simulink model "SarImageFormation"  (Simulink 8.3)
settings: Solver=FixedStepDiscrete  StartTime=0.0  StopTime=0  RelTol=1e-3
model workspace: external: MAT-File SarImageWorkspace.mat (data not in the file)
values from neighbouring files (symbols this model uses):
  m = uicontextmenu('Parent',fig)    [HelperCreateParamTuningUI.m]    (also in HelperMeasureGroupDelay.m = length(p))
  mc = getappdata(uihandle,'midicontrol')    [HelperCreateParamTuningUI.m]
undefined symbols (not defined in the file or in its folder): dkx, fastTimeFilter, ic, jet, k, ku0, kxMin, kxs, magnitude, n, Newton, nInterpSidelobes, nx, Raphson, sRaw, uc, Xc
libraries: dspxfrm3 x4, dspsnks4 x2, dspmathops x2, dspSarDemoLib x2, dspsigops x1, dspmtrx3 x1, dspmisc x1, simulink x1
CloseFcn:
  | if exist('idxout','var') clear idxout; end
  | if exist('sarImage','var') clear sarImage; end
  | sarHandles=findobj('type','figure');
  | for idxh=1:length(sarHandles)
  |     if ~isempty(sarHandles(idxh)) && strcmp(get(sarHandles(idxh), 'UserData'),'SarDemoPlot')
  |        close(sarHandles(idxh));
  |     end
  | end
  | clear sarHandles;
  | clear idxh;
settings Model: FPTRunName=Active  Creator=The MathWorks Inc.  ExtModeAutoUpdateStatusClock=off
settings DataIOCC: SaveOutput=off  SaveTime=off
settings OptimizationCC: InlineParams=on  ExpressionDepthLimit=2147483647  InitFltsAndDblsToZero=on  OptimizeModelRefInitCode=on  LifeSpan=1
settings DebuggingCC: MultiTaskDSMMsg=warning  MultiTaskCondExecSysMsg=none  ParameterPrecisionLossMsg=none  FcnCallInpInsideContextMsg=UseLocalSettings  StrictBusMsg=None
settings HardwareCC: TargetHWDeviceType=32-bit Generic
settings SFSimCC: SimParseCustomCode=off
settings RTWCC: SystemTargetFile=ert.tlc  TemplateMakefile=ert_default_tmf  Description=Real-Time Workshop Embedded Coder (no auto configuration)  ProcessScript=ert_make_rtw_hook  IncludeERTFirstTime=on
settings CodeAppCC: IgnoreCustomStorageClasses=off  CustomSymbolStrType=$N$R$M  InternalIdentifier=Classic
settings ERTTargetCC: TargetFcnLib=ansi_tfl_tmw.mat  MultiwordLength=2048  GenerateSampleERTMain=on  MatFileLogging=on  ERTCustomFileTemplate=example_file_process.tlc  ConvertIfToSwitch=off  SuppressUnreachableDefaultCases=off

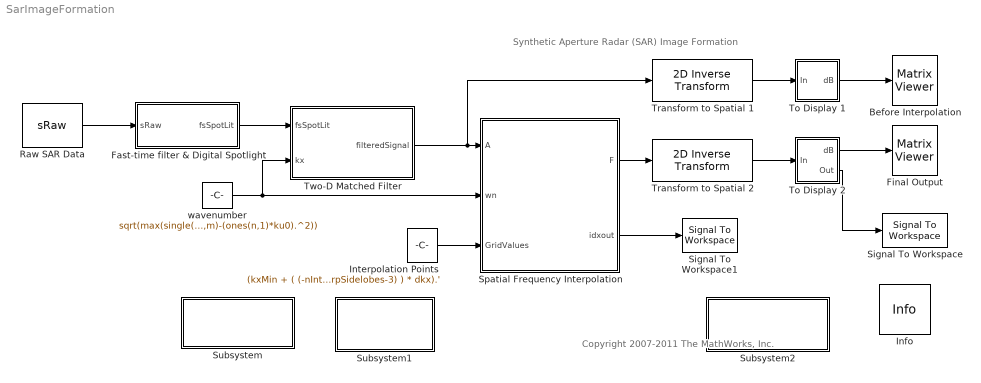
== system SarImageFormation ==
  note: Copyright 2007-2011 The MathWorks, Inc.
  note: Synthetic Aperture Radar (SAR) Image Formation
  Before Interpolation : dspsnks4/Matrix Viewer  ImageParams=off  CMapStr=jet(256)  AxisColorbar=on  AxisParams=off  AxisOrigin=Upper left corner  XLabel=Cross-range  YLabel=Range  ZLabel=Magnitude (dB)  FigPos=[5 300 500 420]  AxisZoom=off
      settings: YMin=0  YMax=60
  Fast-time filter & Digital Spotlight : Subsystem
  Final Output : dspsnks4/Matrix Viewer  ImageParams=off  CMapStr=jet(256)  AxisColorbar=on  AxisParams=off  AxisOrigin=Upper left corner  XLabel=Cross-range  YLabel=Range  ZLabel=Magnitude (dB)  FigPos=[510 300 500 420]  AxisZoom=off
      settings: YMin=0  YMax=60
  Info : dspmisc/Info  SystemSampleTime=-1
  Interpolation Points : Constant  Value=(kxMin + ( (-nInterpSidelobes-2):(nx-nInterpSidelobes-3) ) * dkx).'  VectorParams1D=off  SampleTime=Inf
  Raw SAR Data : Constant  Value=sRaw  VectorParams1D=off  SampleTime=1
  Signal To Workspace : SignalToWorkspace  VariableName=sarImage
      settings: CopyFcn=dspblkcopystw(gcbh);  Save2DSignal=3-D array (concatenate along third dimension)
  Signal To Workspace1 : SignalToWorkspace  VariableName=idxout
      settings: CopyFcn=dspblkcopystw(gcbh);  Save2DSignal=3-D array (concatenate along third dimension)
  Spatial Frequency Interpolation : MATLAB Function  TreatAsAtomicUnit=on
  Subsystem : Subsystem
      settings: OpenFcn=|
      | imagesc(20*log10(fftshift(abs(dspmodelvar(bdroot,'sRaw')))));
      | colorbar;
      | ylabel('Samples');xlabel('Pulses'); title('Spotlight SAR Returns')
      | set(gcf,'UserData','SarDemoPlot');
      mask Display: disp('Display raw\nSAR data (sRaw)')
  Subsystem1 : Subsystem
      settings: OpenFcn=|
      | imagesc(20*log10(abs(dspmodelvar(bdroot,'finalImage').')),[0 60]);
      | colorbar;
      | title('Truth image from MATLAB');
      | set(gcf,'UserData','SarDemoPlot');
      mask Display: disp('Display Truth\nSAR image')
  Subsystem2 : Subsystem
      settings: OpenFcn=|
      | if (exist('idxout','var')),                                        contourf(idxout,50);                                       cb=colorbar;                                                   xlabel('Cross-range');                                     ylabel('Range in source image');                     title('Interpolation Pattern');                            ylabel(cb,'Range in destination image');          clear('cb');
      |      set(gcf,'UserData','SarDemoPlot');            else                                                                     uiwait(errordlg('Data not found in workspace - run demo model.','DSP System Toolbox Demo Error','modal'));    end
      mask Display: disp('Display Interpolation\nPattern (idxout)')
  To Display 1 : Subsystem
  To Display 2 : Subsystem
  Transform to Spatial 1 : dspSarDemoLib/2D Inverse Transform
  Transform to Spatial 2 : dspSarDemoLib/2D Inverse Transform
  Two-D Matched Filter : Subsystem
  wavenumber : Constant  Value=sqrt(max(single(0), 4*(k.').^2*ones(1,m)-(ones(n,1)*ku0).^2))  VectorParams1D=off  SampleTime=Inf
  wires:
  Raw SAR Data/1 -> Fast-time filter & Digital Spotlight/1(sRaw)
  wavenumber/1 -> Spatial Frequency Interpolation/2(wn), Two-D Matched Filter/2(kx)
  To Display 2/1(dB) -> Final Output/1
  Interpolation Points/1 -> Spatial Frequency Interpolation/3(GridValues)
  Fast-time filter & Digital Spotlight/1(fsSpotLit) -> Two-D Matched Filter/1(fsSpotLit)
  Spatial Frequency Interpolation/1(F) -> Transform to Spatial 2/1
  Spatial Frequency Interpolation/2(idxout) -> Signal To Workspace1/1
  Transform to Spatial 2/1 -> To Display 2/1(" In")
  To Display 2/2(Out) -> Signal To Workspace/1
  Two-D Matched Filter/1(filteredSignal) -> Spatial Frequency Interpolation/1(A), Transform to Spatial 1/1
  Transform to Spatial 1/1 -> To Display 1/1(In)
  To Display 1/1(dB) -> Before Interpolation/1

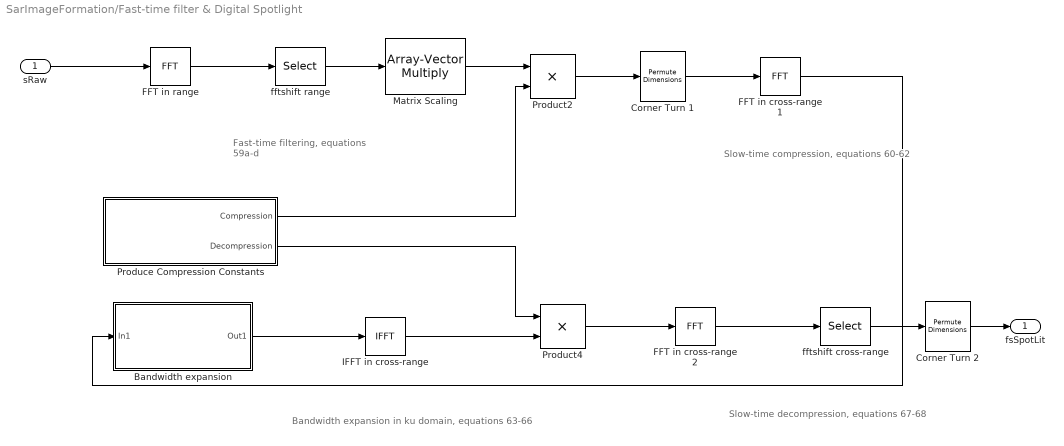
== system SarImageFormation/Fast-time filter & Digital Spotlight ==
  note: Fast-time filtering,
      | equations 59a-d
  note: Slow-time compression, equations 60-62
  note: Bandwidth expansion in ku domain, equations 63-66
  note: Slow-time decompression, equations 67-68
  sRaw : Inport
  Bandwidth expansion : Subsystem
  Corner Turn 1 : PermuteDimensions
  Corner Turn 2 : PermuteDimensions
  FFT in cross-range 1 : dspxfrm3/FFT  CompMethod=Table lookup  TableOpt=NEW  TableOptActive=Speed  BitRevOrder=off  InheritFFTLength=on  FFTLength=64  WrapInput=on  RowConvenienceOn=on  FFTImplementation=Auto  SkipNorm=off  firstCoeffDataTypeStr=Inherit: Same word length as input  firstCoeffLastDataTypeStr=Inherit: Same word length as input  outputMin=[]  outputMax=[]  roundingMode=Floor  overflowMode=off
  FFT in cross-range 2 : dspxfrm3/FFT  CompMethod=Table lookup  TableOpt=NEW  TableOptActive=Speed  BitRevOrder=off  InheritFFTLength=on  FFTLength=64  WrapInput=on  RowConvenienceOn=on  FFTImplementation=Auto  SkipNorm=off  firstCoeffDataTypeStr=Inherit: Same word length as input  firstCoeffLastDataTypeStr=Inherit: Same word length as input  outputMin=[]  outputMax=[]  roundingMode=Floor  overflowMode=off
  FFT in range : dspxfrm3/FFT  CompMethod=Table lookup  TableOpt=NEW  TableOptActive=Speed  BitRevOrder=off  InheritFFTLength=on  FFTLength=64  WrapInput=on  RowConvenienceOn=on  FFTImplementation=Auto  SkipNorm=off  firstCoeffDataTypeStr=Inherit: Same word length as input  firstCoeffLastDataTypeStr=Inherit: Same word length as input  outputMin=[]  outputMax=[]  roundingMode=Floor  overflowMode=off
  IFFT in cross-range : dspxfrm3/IFFT  CompMethod=Table lookup  TableOpt=NEW  TableOptActive=Speed  BitRevOrder=off  cs_in=off  SkipNorm=on  InheritFFTLength=on  FFTLength=64  WrapInput=on  mode=Complex  outSamplingMode=Sample based  RowConvenienceOn=on  FFTImplementation=Auto  firstCoeffDataTypeStr=Inherit: Same word length as input  firstCoeffLastDataTypeStr=Inherit: Same word length as input  outputMin=[]  outputMax=[]  roundingMode=Floor  overflowMode=off
  Matrix Scaling : dspmtrx3/Array-Vector Multiply  mode=Mute  saveAsFlag=0  Dimension=1  V_Source=Dialog parameter  V_VectFromMask=fftshift(fastTimeFilter)  firstCoeffSignedness=Auto  firstCoeffDataTypeStr=Inherit: Same word length as input  firstCoeffLastDataTypeStr=Inherit: Same word length as input  firstCoeffMin=[]  firstCoeffMax=[]  outputSignedness=Auto  outputDataTypeStr=Inherit: Same as product output  outputLastDataTypeStr=Inherit: Same as product output  outputMin=[]  outputMax=[]  accumSignedness=Auto  prodOutputSignedness=Auto  roundingMode=Floor  overflowMode=off
  Produce Compression Constants : Subsystem
  Product2 : Product  RndMeth=Zero
  Product4 : Product  OutDataTypeStr=single  RndMeth=Zero
  fftshift cross-range : Selector  NumberOfDimensions=2  InputPortWidth=3  IndexOptions=Index vector (dialog),Select all  Indices=int32([(m/2+1):m,1:(m/2)]),int32([(m/2+1):m,1:(m/2)])  OutputSizes=1,1
  fftshift range : Selector  NumberOfDimensions=2  InputPortWidth=3  IndexOptions=Index vector (dialog),Select all  Indices=int32([(n/2+1):n,1:(n/2)]),int32([(m/2+1):m,1:(m/2)])  OutputSizes=1,1
  fsSpotLit : Outport
  wires:
  FFT in range/1 -> fftshift range/1
  Product2/1 -> Corner Turn 1/1
  Matrix Scaling/1 -> Product2/1
  Product4/1 -> FFT in cross-range 2/1
  Bandwidth expansion/1(Out1) -> IFFT in cross-range/1
  sRaw/1 -> FFT in range/1
  FFT in cross-range 1/1 -> Bandwidth expansion/1(In1)
  Produce Compression Constants/2(Decompression) -> Product4/1
  IFFT in cross-range/1 -> Product4/2
  Produce Compression Constants/1(Compression) -> Product2/2
  FFT in cross-range 2/1 -> fftshift cross-range/1
  fftshift range/1 -> Matrix Scaling/1
  fftshift cross-range/1 -> Corner Turn 2/1
  Corner Turn 2/1 -> fsSpotLit/1
  Corner Turn 1/1 -> FFT in cross-range 1/1

== system SarImageFormation/Subsystem ==

== system SarImageFormation/Subsystem1 ==

== system SarImageFormation/Subsystem2 ==

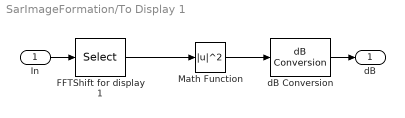
== system SarImageFormation/To Display 1 ==
  In : Inport
  FFTShift for display 1 : Selector  NumberOfDimensions=2  InputPortWidth=3  IndexOptions=Index vector (dialog),Index vector (dialog)  Indices=int32([(n/2+1):n,1:(n/2)]),int32([(m/2+1):m,1:(m/2)])  OutputSizes=1,1
  Math Function : Math  Operator=magnitude^2  SaturateOnIntegerOverflow=on
  dB Conversion : dspmathops/dB Conversion  dBtype=dB  intype=Power  R=1  fuzz=off
  dB : Outport
  wires:
  FFTShift for display 1/1 -> Math Function/1
  Math Function/1 -> dB Conversion/1
  In/1 -> FFTShift for display 1/1
  dB Conversion/1 -> dB/1

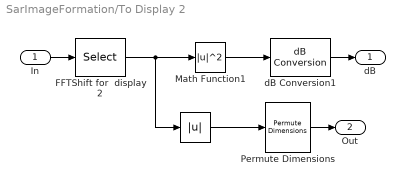
== system SarImageFormation/To Display 2 ==
  " In" : Inport
  " " : Abs
  FFTShift for  display 2 : Selector  NumberOfDimensions=2  InputPortWidth=3  IndexOptions=Index vector (dialog),Index vector (dialog)  Indices=int32([(nx/2+1):nx,1:(nx/2)]),int32([(m/2+1):m,1:(m/2)])  OutputSizes=1,1
  Math Function1 : Math  Operator=magnitude^2  SaturateOnIntegerOverflow=on
  Permute Dimensions : PermuteDimensions
  dB Conversion1 : dspmathops/dB Conversion  dBtype=dB  intype=Power  R=1  fuzz=off
  dB : Outport
  Out : Outport  Port=2
  wires:
  Math Function1/1 -> dB Conversion1/1
  " "/1 -> Permute Dimensions/1
  FFTShift for  display 2/1 -> Math Function1/1, " "/1
  " In"/1 -> FFTShift for  display 2/1
  dB Conversion1/1 -> dB/1
  Permute Dimensions/1 -> Out/1

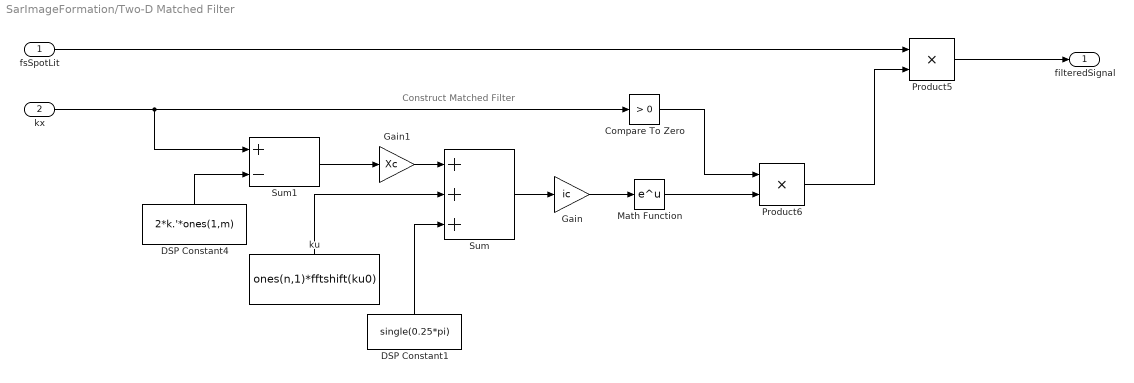
== system SarImageFormation/Two-D Matched Filter ==
  note: Construct Matched Filter
  fsSpotLit : Inport
  kx : Inport  Port=2
  Compare To Zero : simulink/Logic and Bit Operations/Compare To Zero  relop=>  OutDataTypeStr=uint8  ZeroCross=off
  DSP Constant1 : Constant  Value=single(0.25*pi)  VectorParams1D=off  OutDataTypeStr=single  SampleTime=Inf
  DSP Constant4 : Constant  Value=2*k.'*ones(1,m)  VectorParams1D=off  SampleTime=Inf
  Gain : Gain  Gain=ic
  Gain1 : Gain  Gain=Xc
  Math Function : Math  SaturateOnIntegerOverflow=on
  Product5 : Product  RndMeth=Zero
  Product6 : Product  RndMeth=Zero
  Sum : Sum  Inputs=+++
  Sum1 : Sum  Inputs=+-
  ku : Constant  Value=ones(n,1)*fftshift(ku0)  VectorParams1D=off  SampleTime=Inf
  filteredSignal : Outport
  wires:
  kx/1 -> Compare To Zero/1, Sum1/1
  Sum/1 -> Gain/1
  Product5/1 -> filteredSignal/1
  Compare To Zero/1 -> Product6/1
  Math Function/1 -> Product6/2
  Product6/1 -> Product5/2
  fsSpotLit/1 -> Product5/1
  ku/1 -> Sum/2
  DSP Constant1/1 -> Sum/3
  Gain/1 -> Math Function/1
  Sum1/1 -> Gain1/1
  Gain1/1 -> Sum/1
  DSP Constant4/1 -> Sum1/2

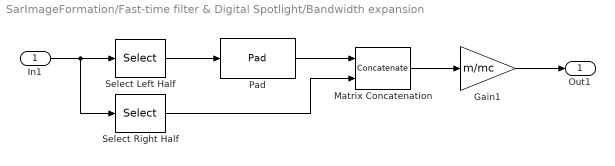
== system SarImageFormation/Fast-time filter & Digital Spotlight/Bandwidth expansion ==
  In1 : Inport
  Gain1 : Gain  Gain=m/mc  OutDataTypeStr=Inherit: Same as input
  Matrix Concatenation : Concatenate  Mode=Multidimensional array
  Pad : dspsigops/Pad  padAlong=Columns  dimsToPad=1  valSrc=Specify via dialog  padVal=0  spec=Output size  padNumOutRowsSpecMethod=User-specified  numOutRows=(m-mc)+(mc/2)  padNumOutColsSpecMethod=User-specified  numOutCols=(m-mc)+(mc/2)  isVarDimsMode=off  padBeginning=0  padEnd=0  outSizeMode=User-specified  outSize=1  padSigAt=End  trunc_flag=None  roundingMode=Floor  overflowMode=off  truncOrWrapMode=Truncate  wrap_flag=None
  Select Left Half : Selector  NumberOfDimensions=2  InputPortWidth=3  IndexOptions=Index vector (dialog),Select all  Indices=int32(1:(mc/2)),int32(1:(mc/2))  OutputSizes=1,1
  Select Right Half : Selector  NumberOfDimensions=2  InputPortWidth=3  IndexOptions=Index vector (dialog),Select all  Indices=int32((mc/2+1):mc),int32((mc/2+1):mc)  OutputSizes=1,1
  Out1 : Outport
  wires:
  In1/1 -> Select Right Half/1, Select Left Half/1
  Select Left Half/1 -> Pad/1
  Pad/1 -> Matrix Concatenation/1
  Select Right Half/1 -> Matrix Concatenation/2
  Matrix Concatenation/1 -> Gain1/1
  Gain1/1 -> Out1/1

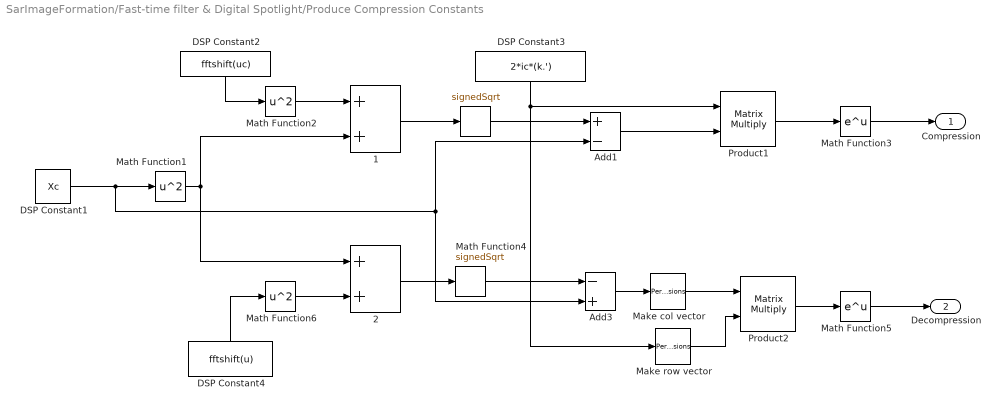
== system SarImageFormation/Fast-time filter & Digital Spotlight/Produce Compression Constants ==
  " " : Sqrt  Operator=signedSqrt  AlgorithmType=Newton-Raphson  SaturateOnIntegerOverflow=on
  " 1" : Sum
  " 2" : Sum
  Add1 : Sum  Inputs=+-
  Add3 : Sum  Inputs=-+
  DSP Constant1 : Constant  Value=Xc  VectorParams1D=off  SampleTime=Inf
  DSP Constant2 : Constant  Value=fftshift(uc)  VectorParams1D=off  SampleTime=Inf
  DSP Constant3 : Constant  Value=2*ic*(k.')  VectorParams1D=off  SampleTime=Inf
  DSP Constant4 : Constant  Value=fftshift(u)  VectorParams1D=off  SampleTime=Inf
  Make col vector : PermuteDimensions
  Make row vector : PermuteDimensions
  Math Function1 : Math  Operator=square  SaturateOnIntegerOverflow=on
  Math Function2 : Math  Operator=square  SaturateOnIntegerOverflow=on
  Math Function3 : Math  SaturateOnIntegerOverflow=on
  Math Function4 : Sqrt  Operator=signedSqrt  AlgorithmType=Newton-Raphson  SaturateOnIntegerOverflow=on
  Math Function5 : Math  SaturateOnIntegerOverflow=on
  Math Function6 : Math  Operator=square  SaturateOnIntegerOverflow=on
  Product1 : Product  Multiplication=Matrix(*)  RndMeth=Zero
  Product2 : Product  Multiplication=Matrix(*)  OutDataTypeStr=single  RndMeth=Zero  InputSameDT=on
  Compression : Outport
  Decompression : Outport  Port=2
  wires:
  Math Function1/1 -> " 1"/2, " 2"/1
  " 1"/1 -> " "/1
  DSP Constant2/1 -> Math Function2/1
  Add1/1 -> Product1/2
  Product1/1 -> Math Function3/1
  " 2"/1 -> Math Function4/1
  Add3/1 -> Make col vector/1
  DSP Constant4/1 -> Math Function6/1
  Product2/1 -> Math Function5/1
  Math Function6/1 -> " 2"/2
  DSP Constant1/1 -> Math Function1/1, Add1/2, Add3/2
  DSP Constant3/1 -> Product1/1, Make row vector/1
  Math Function4/1 -> Add3/1
  " "/1 -> Add1/1
  Math Function3/1 -> Compression/1
  Math Function5/1 -> Decompression/1
  Math Function2/1 -> " 1"/1
  Make col vector/1 -> Product2/1
  Make row vector/1 -> Product2/2

== matlab function Spatial Frequency Interpolation ==
  data: A input double; wn input double; GridValues input double; dkx parameter double; kxs parameter double; F output double; idxout output double
function [F,idxout] = SpatialInterpolate(A, wn, GridValues, ...
    dkx, kxs)

nInterpSidelobes = 8;

nx = size(GridValues,1); % Final image output rows

[n, m] = size(wn); % Size of spatial frequency data
offset = 1:(2*nInterpSidelobes-1);
p = length(offset);


rowidx = round((wn - GridValues(1))/dkx) - nInterpSidelobes;
idxout = single(zeros(n,m));
SliceRange = single(zeros(n,m));
F = single(complex(zeros(nx, m),zeros(nx,m)));

% Each row of the matrix influences 'p' other rows, one for each sidelobe of
% the interpolation function
for iz = 1:p
    
    % Use the base row index and the index of this sidelobe to find
    % the index of the row that each point influences
    idxout = rowidx + offset(iz);
    % Compute the m by n image corresponding to this sidelobe
    for ix = 1:n
        for iy = 1:m
            % SliceRange is a translation of the index into corresponding
            % coordinates, used to calculate the windowing functions
            SliceRange(ix, iy) = GridValues(idxout(ix,iy)) - wn(ix, iy);
        end
    end
    
    % Compute interpolating windows from the slice values
    snc = sinc(SliceRange/dkx);
    ham = 0.54 + 0.46*cos( SliceRange *(pi/kxs));

    % Compute interpolated signal spectrum
    for ix = 1:n
        for iy = 1:m
            F(idxout(ix,iy), iy) = F(idxout(ix,iy), iy) + A(ix,iy)*snc(ix,iy)*ham(ix,iy);
        end
    end
end

function y = sinc(x)
% function y = sinc(A, ridx)
% sin(x)/x

y = x;
for ix = 1:numel(x)
    if x(ix)==0
        y(ix)=1;
    else
        y(ix) = sin(pi*x(ix))/(pi*x(ix));
    end
end
